simulink model "evitar_choque_funcional"  (R2023b)
settings: Solver=FixedStepAuto  StartTime=0.0  StopTime=inf  RelTol=1e-3  EnableMultiTasking=on
settings Model: ExtModeTrigDuration=2  Creator=Usuario_UMA  LastModifiedBy=juana
settings OptimizationCC: EnhancedBackFolding=on  PassReuseOutputArgsAs=Individual arguments  ZeroExternalMemoryAtStartup=off  ZeroInternalMemoryAtStartup=off  MaxStackSize=64  OptimizeBlockOrder=speed  DifferentSizesBufferReuse=on  OptimizationCustomize=off  EfficientTunableParamExpr=on
settings DebuggingCC: ParameterTunabilityLossMsg=error
settings HardwareCC: ProdBitPerInt=16  ProdBitPerPointer=16  ProdBitPerSizeT=16  ProdBitPerPtrDiffT=16  ProdLargestAtomicFloat=None  ProdWordSize=8  ProdHWDeviceType=Atmel->AVR  UseEmbeddedCoderFeatures=off  UseSimulinkCoderFeatures=off
settings SFSimCC: MATLABDynamicMemAlloc=off
settings RTWCC: Description=Embedded Coder  SystemTargetFile=ert.tlc  HardwareBoard=Arduino Mega 2560  TemplateMakefile=ert_default_tmf  Toolchain=Arduino AVR  BuildConfiguration=Faster Runs
settings CodeAppCC: ForceParamTrailComments=on  IgnoreCustomStorageClasses=off  OperatorAnnotations=on  SimulinkDataObjDesc=on  SFDataObjDesc=on  MangleLength=10  InsertBlockDesc=on
settings ERTTargetCC: SupportContinuousTime=on  SupportNonInlinedSFcns=on  SupportVariableSizeSignals=on  ExtModeTransport=3  ExtModeStaticAlloc=on  ExtModeAutomaticAllocSize=off  ExtModeStaticAllocSize=2048  ExtModeMexFile=ext_xcp  ExtModeIntrfLevel=Level2 - Open

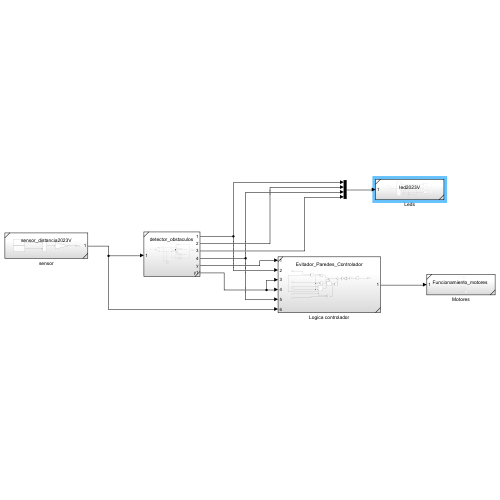
[thumbnail: Simulink's stored preview of the top-level diagram]
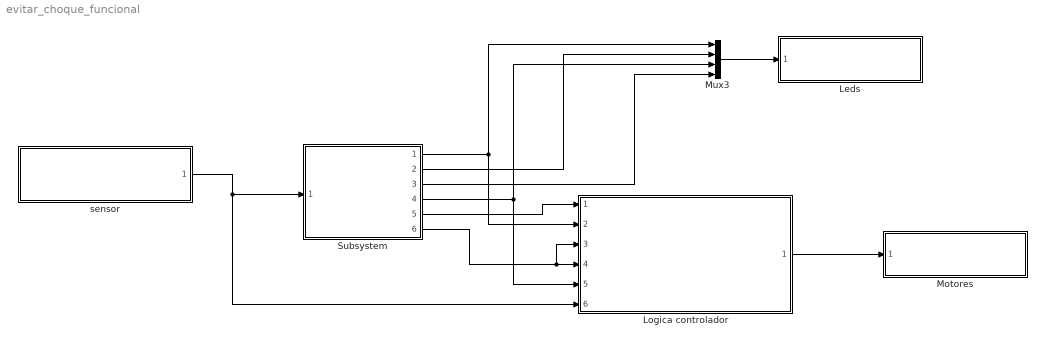
== system evitar_choque_funcional ==
  Leds : Subsystem  ReferencedSubsystem=led2023V
  Logica controlador : Subsystem  ReferencedSubsystem=Evitador_Paredes_Controlador
  Motores : Subsystem  ReferencedSubsystem=Funcionamiento_motores
  Mux3 : Mux
  Subsystem : Subsystem  ReferencedSubsystem=detector_obstaculos
  sensor : Subsystem  ReferencedSubsystem=sensor_distancia2023V
  wires:
  sensor/1 -> Subsystem/1, Logica controlador/6
  Mux3/1 -> Leds/1
  Logica controlador/1 -> Motores/1
  Subsystem/6 -> Logica controlador/3, Logica controlador/4
  Subsystem/1 -> Mux3/1, Logica controlador/2
  Subsystem/4 -> Mux3/3, Logica controlador/5
  Subsystem/2 -> Mux3/2
  Subsystem/3 -> Mux3/4
  Subsystem/5 -> Logica controlador/1
